simulink model "blocos"  (R2013a)
settings: Solver=ode45  StartTime=0.0  StopTime=3  RelTol=1e-3
values from neighbouring files (symbols this model uses):
  alpha = (Lms+Lls)    (= 0.11)    [Sugestao de estrutura de programa.m]
  beta = (Llr+Lms)    (= 0.11)    [Sugestao de estrutura de programa.m]
  Bm = dl    (= 0.0001)    [Sugestao de estrutura de programa.m]
  f = 60    [Sugestao de estrutura de programa.m]
  J = Jl    (= 0.002)    [Sugestao de estrutura de programa.m]
  Jl = 0.002    [Sugestao de estrutura de programa.m]
  Llr = 0.01    [Sugestao de estrutura de programa.m]
  Lls = 0.01    [Sugestao de estrutura de programa.m]
  Lms = 0.1    [Sugestao de estrutura de programa.m]
  P = 2    [Sugestao de estrutura de programa.m]
  polos = 2    [Sugestao de estrutura de programa.m]
  rrs = 1    [Sugestao de estrutura de programa.m]
  rs = 0.8    [Sugestao de estrutura de programa.m]
  thetar = 0.0    (= 0)    [Sugestao de estrutura de programa.m]
  U = 220    [Sugestao de estrutura de programa.m]
undefined symbols (not defined in the file or in its folder): i
settings Model: Creator=Charles  LastModifiedBy=Charles

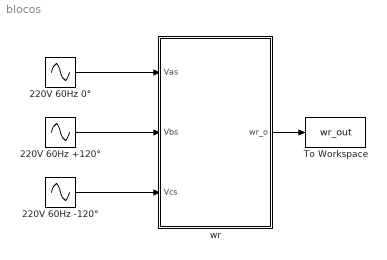
== system blocos ==
  220V 60Hz +120° : Sin  Amplitude=220  Frequency=377  Phase=2.0944  SampleTime=0
  220V 60Hz -120° : Sin  Amplitude=220  Frequency=377  Phase=-2.0944  SampleTime=0
  220V 60Hz 0° : Sin  Amplitude=220  Frequency=377  SampleTime=0
  To Workspace : ToWorkspace  VariableName=wr_out  SampleTime=-1  SaveFormat=Timeseries
  wr : Subsystem
  wires:
  220V 60Hz 0°/1 -> wr/1(Vas)
  wr/1(wr_o) -> To Workspace/1
  220V 60Hz +120°/1 -> wr/2(Vbs)
  220V 60Hz -120°/1 -> wr/3(Vcs)

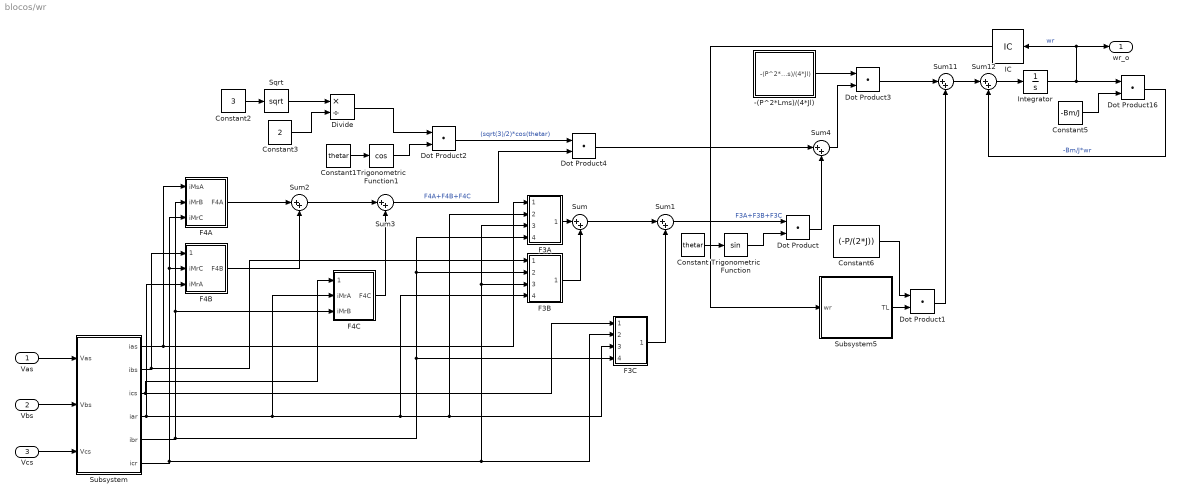
== system blocos/wr ==
  Vas : Inport
  Vbs : Inport  Port=2
  Vcs : Inport  Port=3
  -(P^2*Lms)/(4*Jl) : Subsystem
  Constant : Constant  Value=thetar
  Constant1 : Constant  Value=thetar
  Constant2 : Constant  Value=3
  Constant3 : Constant  Value=2
  Constant5 : Constant  Value=-Bm/J
  Constant6 : Constant  Value=(-P/(2*J))
  Divide : Product  Inputs=*/
  Dot Product{,1..4,16} (6 alike) : DotProduct  InputSameDT=on  OutDataTypeStr=Inherit: Inherit via internal rule
  F3A : Subsystem
  F3B : Subsystem
  F3C : Subsystem
  F4A : Subsystem
  F4B : Subsystem
  F4C : Subsystem
  IC : InitialCondition  Value=0.000001
  Integrator : Integrator
  Sqrt : Sqrt  SaturateOnIntegerOverflow=on
  Subsystem : Subsystem
  Subsystem5 : Subsystem
  Sum{,1..4,11..12} (7 alike) : Sum  Inputs=|++
  Trigonometric Function : Trigonometry
  Trigonometric Function1 : Trigonometry  Operator=cos
  wr_o : Outport
  wires:
  Dot Product16/1 -> Sum12/2  "-Bm/J*wr"
  Integrator/1 -> wr_o/1, IC/1, Dot Product16/1  "wr"
  Sum11/1 -> Sum12/1
  Constant5/1 -> Dot Product16/2
  Subsystem/3(ics) -> F3C/1(iMsC), F4C/1(iMsC)
  Subsystem/4(iar) -> F3C/3(iMrA), F3A/2(iMrA), F3B/4(iMrA), F4C/2(iMrA), F4B/3(iMrA)
  Subsystem/5(ibr) -> F3C/4(iMrB), F3B/2(iMrB), F3A/4(iMrB), F4C/3(iMrB), F4A/2(iMrB)
  Vbs/1 -> Subsystem/2(Vbs)
  Vcs/1 -> Subsystem/3(Vcs)
  Subsystem/2(ibs) -> F3B/1(iMsB), F4B/1(iMsB)
  Subsystem/6(icr) -> F3C/2(iMrC), F3B/3(iMrC), F3A/3(iMrC), F4B/2(iMrC), F4A/3(iMrC)
  Subsystem/1(ias) -> F3A/1(iMsA), F4A/1(iMsA)
  F4C/1(F4C) -> Sum3/2
  Sum3/1 -> Dot Product4/2  "F4A+F4B+F4C"
  Divide/1 -> Dot Product2/1
  Constant1/1 -> Trigonometric Function1/1
  F3B/1(F3B) -> Sum/2
  Trigonometric Function/1 -> Dot Product/2
  Constant2/1 -> Sqrt/1
  Sum1/1 -> Dot Product/1  "F3A+F3B+F3C"
  Dot Product4/1 -> Sum4/1
  F4B/1(F4B) -> Sum2/2
  F3C/1(F3C) -> Sum1/2
  Dot Product/1 -> Sum4/2
  Trigonometric Function1/1 -> Dot Product2/2
  Sum/1 -> Sum1/1
  Sqrt/1 -> Divide/1
  F4A/1(F4A) -> Sum2/1
  Sum2/1 -> Sum3/1
  Constant3/1 -> Divide/2
  Dot Product2/1 -> Dot Product4/1  "(sqrt(3)/2)*cos(thetar)"
  Dot Product3/1 -> Sum11/1
  -(P^2*Lms)/(4*Jl)/1(-(P^2*Lms)/(4*Jl)) -> Dot Product3/1
  Sum4/1 -> Dot Product3/2
  F3A/1(F3A) -> Sum/1
  Constant/1 -> Trigonometric Function/1
  Vas/1 -> Subsystem/1(Vas)
  Subsystem5/1(TL) -> Dot Product1/2
  Dot Product1/1 -> Sum11/2
  Constant6/1 -> Dot Product1/1
  Sum12/1 -> Integrator/1
  IC/1 -> Subsystem5/1(wr)

== system blocos/wr/-(P^2*Lms)//(4*Jl) ==
  Constant : Constant  Value=P
  Constant1 : Constant  Value=-Lms
  Constant2 : Constant  Value=4*Jl
  Divide : Product  Inputs=*/
  Dot Product : DotProduct  InputSameDT=on  OutDataTypeStr=Inherit: Inherit via internal rule
  Dot Product1 : DotProduct  InputSameDT=on  OutDataTypeStr=Inherit: Inherit via internal rule
  -(P^2*Lms)/(4*Jl) : Outport
  wires:
  Divide/1 -> -(P^2*Lms)/(4*Jl)/1  "-(P^2*Lms)/(4*Jl)"
  Constant2/1 -> Divide/2
  Dot Product1/1 -> Divide/1  "-P^2*Lms"
  Dot Product/1 -> Dot Product1/1  "P^2"
  Constant1/1 -> Dot Product1/2
  Constant/1 -> Dot Product/2, Dot Product/1

== system blocos/wr/F3A ==
  iMsA : Inport
  iMrA : Inport  Port=2
  iMrC : Inport  Port=3
  iMrB : Inport  Port=4
  Constant : Constant  Value=-0.5
  Dot Product : DotProduct  InputSameDT=on  OutDataTypeStr=Inherit: Inherit via internal rule
  Dot Product1 : DotProduct  InputSameDT=on  OutDataTypeStr=Inherit: Inherit via internal rule
  Dot Product2 : DotProduct  InputSameDT=on  OutDataTypeStr=Inherit: Inherit via internal rule
  Sum : Sum  Inputs=|++
  Sum1 : Sum  Inputs=|++
  F3A : Outport
  wires:
  iMrB/1 -> Dot Product/1
  Sum1/1 -> Dot Product2/1  "iMrA-0.5*iMrB-0.5*iMrC"
  iMrA/1 -> Sum1/2
  Dot Product2/1 -> F3A/1
  iMrC/1 -> Dot Product1/1
  Constant/1 -> Dot Product/2, Dot Product1/2
  Dot Product/1 -> Sum/1  "-0.5*iMrB"
  Sum/1 -> Sum1/1  "-0.5*iMrB-0.5*iMrC"
  iMsA/1 -> Dot Product2/2
  Dot Product1/1 -> Sum/2  "-0.5*iMrC"

== system blocos/wr/F3B ==
  iMsB : Inport
  iMrB : Inport  Port=2
  iMrC : Inport  Port=3
  iMrA : Inport  Port=4
  Constant : Constant  Value=-0.5
  Dot Product : DotProduct  InputSameDT=on  OutDataTypeStr=Inherit: Inherit via internal rule
  Dot Product1 : DotProduct  InputSameDT=on  OutDataTypeStr=Inherit: Inherit via internal rule
  Dot Product2 : DotProduct  InputSameDT=on  OutDataTypeStr=Inherit: Inherit via internal rule
  Sum : Sum  Inputs=|++
  Sum1 : Sum  Inputs=|++
  F3B : Outport
  wires:
  iMrA/1 -> Dot Product/1
  Sum1/1 -> Dot Product2/1  "iMrB-0.5*iMrA-0.5*iMrC"
  iMrB/1 -> Sum1/2
  Dot Product2/1 -> F3B/1
  iMrC/1 -> Dot Product1/1
  Constant/1 -> Dot Product/2, Dot Product1/2
  Dot Product/1 -> Sum/1  "-0.5*iMrA"
  Sum/1 -> Sum1/1  "-0.5*iMrA-0.5*iMrC"
  iMsB/1 -> Dot Product2/2
  Dot Product1/1 -> Sum/2  "-0.5*iMrC"

== system blocos/wr/F3C ==
  iMsC : Inport
  iMrC : Inport  Port=2
  iMrA : Inport  Port=3
  iMrB : Inport  Port=4
  Constant : Constant  Value=-0.5
  Dot Product : DotProduct  InputSameDT=on  OutDataTypeStr=Inherit: Inherit via internal rule
  Dot Product1 : DotProduct  InputSameDT=on  OutDataTypeStr=Inherit: Inherit via internal rule
  Dot Product2 : DotProduct  InputSameDT=on  OutDataTypeStr=Inherit: Inherit via internal rule
  Sum : Sum  Inputs=|++
  Sum1 : Sum  Inputs=|++
  F3C : Outport
  wires:
  iMrB/1 -> Dot Product/1
  Sum1/1 -> Dot Product2/1  "iMrC-0.5*iMrB-0.5*iMrA"
  iMrC/1 -> Sum1/2
  Dot Product2/1 -> F3C/1
  iMrA/1 -> Dot Product1/1
  Constant/1 -> Dot Product/2, Dot Product1/2
  Dot Product/1 -> Sum/1  "-0.5*iMrB"
  Sum/1 -> Sum1/1  "-0.5*iMrB-0.5*iMrA"
  iMsC/1 -> Dot Product2/2
  Dot Product1/1 -> Sum/2  "-0.5*iMrA"

== system blocos/wr/F4A ==
  iMsA : Inport
  iMrB : Inport  Port=2
  iMrC : Inport  Port=3
  Dot Product : DotProduct  InputSameDT=on  OutDataTypeStr=Inherit: Inherit via internal rule
  Subtract1 : Sum  Inputs=+-
  F4A : Outport
  wires:
  Subtract1/1 -> Dot Product/2
  iMrC/1 -> Subtract1/2
  iMrB/1 -> Subtract1/1
  Dot Product/1 -> F4A/1
  iMsA/1 -> Dot Product/1

== system blocos/wr/F4B ==
  iMsB : Inport
  iMrC : Inport  Port=2
  iMrA : Inport  Port=3
  Dot Product : DotProduct  InputSameDT=on  OutDataTypeStr=Inherit: Inherit via internal rule
  Subtract1 : Sum  Inputs=+-
  F4B : Outport
  wires:
  Subtract1/1 -> Dot Product/2
  iMrA/1 -> Subtract1/2
  iMrC/1 -> Subtract1/1
  Dot Product/1 -> F4B/1
  iMsB/1 -> Dot Product/1

== system blocos/wr/F4C ==
  iMsC : Inport
  iMrA : Inport  Port=2
  iMrB : Inport  Port=3
  Dot Product : DotProduct  InputSameDT=on  OutDataTypeStr=Inherit: Inherit via internal rule
  Subtract1 : Sum  Inputs=+-
  F4C : Outport
  wires:
  Subtract1/1 -> Dot Product/2
  iMrB/1 -> Subtract1/2
  iMrA/1 -> Subtract1/1
  Dot Product/1 -> F4C/1
  iMsC/1 -> Dot Product/1

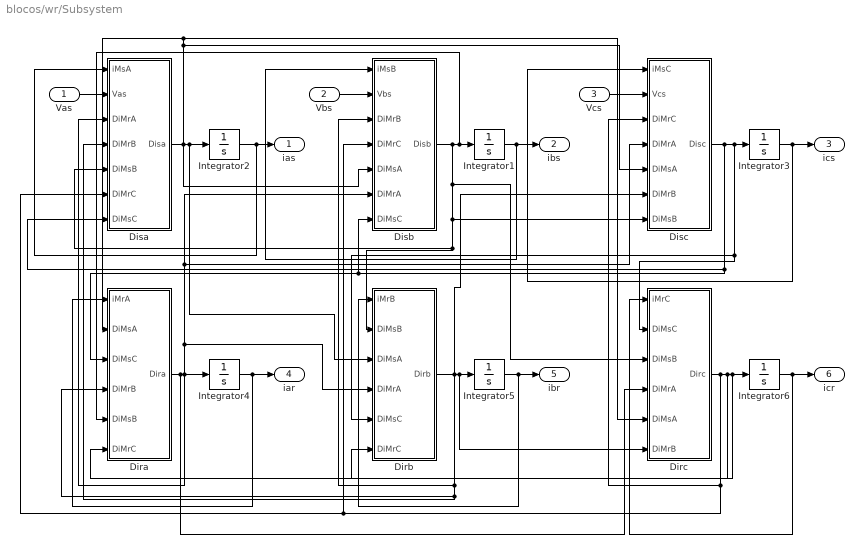
== system blocos/wr/Subsystem ==
  Vas : Inport
  Vbs : Inport  Port=2
  Vcs : Inport  Port=3
  Dira : Subsystem
  Dirb : Subsystem
  Dirc : Subsystem
  Disa : Subsystem
  Disb : Subsystem
  Disc : Subsystem
  Integrator{1..6} (6 alike) : Integrator
  ias : Outport
  ibs : Outport  Port=2
  ics : Outport  Port=3
  iar : Outport  Port=4
  ibr : Outport  Port=5
  icr : Outport  Port=6
  wires:
  Integrator2/1 -> Disa/1(iMsA), ias/1
  Disa/1(Disa) -> Dira/2(DiMsA), Dirc/5(DiMsA), Disc/5(DiMsA), Disb/5(DiMsA), Dirb/3(DiMsA), Integrator2/1
  Integrator1/1 -> Disb/1(iMsB), ibs/1
  Disb/1(Disb) -> Dirc/3(DiMsB), Dirb/2(DiMsB), Disa/5(DiMsB), Disc/7(DiMsB), Dira/5(DiMsB), Integrator1/1
  Integrator3/1 -> Disc/1(iMsC), ics/1
  Disc/1(Disc) -> Dira/3(DiMsC), Disb/7(DiMsC), Disa/7(DiMsC), Dirc/2(DiMsC), Dirb/5(DiMsC), Integrator3/1
  Integrator4/1 -> Dira/1(iMrA), iar/1
  Dira/1(Dira) -> Dirc/4(DiMrA), Dirb/4(DiMrA), Disc/4(DiMrA), Disb/6(DiMrA), Disa/3(DiMrA), Integrator4/1
  Integrator5/1 -> Dirb/1(iMrB), ibr/1
  Dirb/1(Dirb) -> Dira/4(DiMrB), Disa/4(DiMrB), Disb/3(DiMrB), Disc/6(DiMrB), Dirc/6(DiMrB), Integrator5/1
  Integrator6/1 -> Dirc/1(iMrC), icr/1
  Dirc/1(Dirc) -> Disc/3(DiMrC), Disb/4(DiMrC), Disa/6(DiMrC), Dirb/6(DiMrC), Dira/6(DiMrC), Integrator6/1
  Vas/1 -> Disa/2(Vas)
  Vbs/1 -> Disb/2(Vbs)
  Vcs/1 -> Disc/2(Vcs)

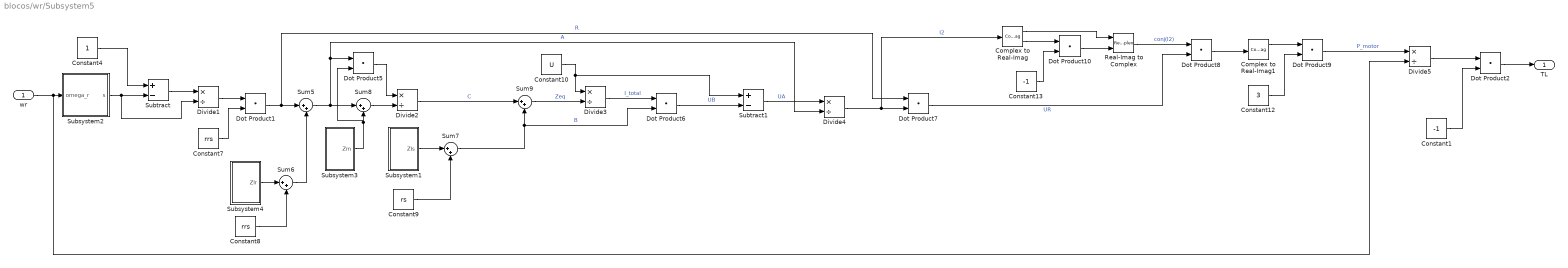
== system blocos/wr/Subsystem5 ==
  wr : Inport
  Complex to Real-Imag : ComplexToRealImag
  Complex to Real-Imag1 : ComplexToRealImag
  Constant1 : Constant  Value=-1
  Constant10 : Constant  Value=U
  Constant12 : Constant  Value=3
  Constant13 : Constant  Value=-1
  Constant4 : Constant
  Constant7 : Constant  Value=rrs
  Constant8 : Constant  Value=rrs
  Constant9 : Constant  Value=rs
  Divide{1..5} (5 alike) : Product  Inputs=*/
  Dot Product{1..2,5..10} (8 alike) : DotProduct  InputSameDT=on  OutDataTypeStr=Inherit: Inherit via internal rule
  Real-Imag to Complex : RealImagToComplex
  Subsystem1 : Subsystem
  Subsystem2 : Subsystem
  Subsystem3 : Subsystem
  Subsystem4 : Subsystem
  Subtract : Sum  Inputs=+-
  Subtract1 : Sum  Inputs=+-
  Sum{5..9} (5 alike) : Sum  Inputs=|++
  TL : Outport
  wires:
  Constant7/1 -> Dot Product1/2
  Dot Product1/1 -> Dot Product7/1, Sum5/1  "R"
  Divide1/1 -> Dot Product1/1
  Constant4/1 -> Subtract/1
  Subtract/1 -> Divide1/1
  Subsystem2/1(s) -> Divide1/2, Subtract/2
  wr/1 -> Divide5/2, Subsystem2/1(omega_r)
  Constant10/1 -> Subtract1/1, Divide3/1
  Subsystem3/1(Zm) -> Dot Product5/2, Sum8/2
  Divide3/1 -> Dot Product6/1  "I_total"
  Subtract1/1 -> Divide4/1  "UA"
  Sum8/1 -> Divide2/2
  Sum6/1 -> Sum5/2
  Constant8/1 -> Sum6/2
  Sum5/1 -> Divide4/2, Dot Product5/1, Sum8/1  "A"
  Divide4/1 -> Complex to Real-Imag/1, Dot Product7/2  "I2"
  Subsystem4/1(Zlr) -> Sum6/1
  Divide2/1 -> Sum9/1  "C"
  Dot Product5/1 -> Divide2/1
  Dot Product7/1 -> Dot Product8/2  "UR"
  Subsystem1/1(Zls) -> Sum7/1
  Constant9/1 -> Sum7/2
  Dot Product6/1 -> Subtract1/2  "UB"
  Sum7/1 -> Dot Product6/2, Sum9/2  "B"
  Sum9/1 -> Divide3/2  "Zeq"
  Constant12/1 -> Dot Product9/2
  Complex to Real-Imag/2 -> Dot Product10/1
  Complex to Real-Imag1/1 -> Dot Product9/1
  Dot Product9/1 -> Divide5/1  "P_motor"
  Complex to Real-Imag/1 -> Real-Imag to Complex/1
  Dot Product10/1 -> Real-Imag to Complex/2
  Constant13/1 -> Dot Product10/2
  Real-Imag to Complex/1 -> Dot Product8/1  "conj(I2)"
  Dot Product8/1 -> Complex to Real-Imag1/1
  Constant1/1 -> Dot Product2/2
  Divide5/1 -> Dot Product2/1
  Dot Product2/1 -> TL/1

== system blocos/wr/Subsystem/Dira ==
  iMrA : Inport
  DiMsA : Inport  Port=2
  DiMsC : Inport  Port=3
  DiMrB : Inport  Port=4
  DiMsB : Inport  Port=5
  DiMrC : Inport  Port=6
  1/beta : Constant  Value=1/beta
  Constant : Constant  Value=-rrs
  Dot Product : DotProduct  InputSameDT=on  OutDataTypeStr=Inherit: Inherit via internal rule
  Dot Product1 : DotProduct  InputSameDT=on  OutDataTypeStr=Inherit: Inherit via internal rule
  F1A1 : Subsystem
  F2A 1 : Subsystem
  Sum1 : Sum  Inputs=|++
  Sum2 : Sum  Inputs=|++
  Dira : Outport
  wires:
  Dot Product/1 -> Sum1/1  "-rrs*iMrA"
  iMrA/1 -> Dot Product/1
  Constant/1 -> Dot Product/2
  Sum1/1 -> Sum2/1  "-rrs*iMrA+F1Ar"
  Sum2/1 -> Dot Product1/1  "-rrs*iMrA+F1Ar+F2Ar"
  F2A 1/1(F2Ar) -> Sum2/2
  DiMrC/1 -> F1A1/2(DiMrC)
  F1A1/1(F1Ar) -> Sum1/2
  DiMrB/1 -> F1A1/1(DiMrB)
  1/beta/1 -> Dot Product1/2
  DiMsB/1 -> F2A 1/3(DiMsB)
  Dot Product1/1 -> Dira/1
  DiMsC/1 -> F2A 1/2(DiMsC)
  DiMsA/1 -> F2A 1/1(DiMsA)

== system blocos/wr/Subsystem/Dirb ==
  iMrB : Inport
  DiMsB : Inport  Port=2
  DiMsA : Inport  Port=3
  DiMrA : Inport  Port=4
  DiMsC : Inport  Port=5
  DiMrC : Inport  Port=6
  1/beta : Constant  Value=1/beta
  Constant : Constant  Value=-rrs
  Dot Product : DotProduct  InputSameDT=on  OutDataTypeStr=Inherit: Inherit via internal rule
  Dot Product1 : DotProduct  InputSameDT=on  OutDataTypeStr=Inherit: Inherit via internal rule
  F1A1 : Subsystem
  F2A 1 : Subsystem
  Sum1 : Sum  Inputs=|++
  Sum2 : Sum  Inputs=|++
  Dirb : Outport
  wires:
  Dot Product/1 -> Sum1/1  "-rrs*iMrB"
  iMrB/1 -> Dot Product/1
  Constant/1 -> Dot Product/2
  Sum1/1 -> Sum2/1  "-rrs*iMrB+F1Br"
  Sum2/1 -> Dot Product1/1  "-rrs*iMrB+F1Br+F2Br"
  F2A 1/1(F2Br) -> Sum2/2
  DiMrC/1 -> F1A1/2(DiMrC)
  F1A1/1(F1Br) -> Sum1/2
  DiMrA/1 -> F1A1/1(DiMrA)
  1/beta/1 -> Dot Product1/2
  DiMsC/1 -> F2A 1/3(DiMsC)
  Dot Product1/1 -> Dirb/1
  DiMsA/1 -> F2A 1/2(DiMsA)
  DiMsB/1 -> F2A 1/1(DiMsB)

== system blocos/wr/Subsystem/Dirc ==
  iMrC : Inport
  DiMsC : Inport  Port=2
  DiMsB : Inport  Port=3
  DiMrA : Inport  Port=4
  DiMsA : Inport  Port=5
  DiMrB : Inport  Port=6
  1/beta : Constant  Value=1/beta
  Constant : Constant  Value=-rrs
  Dot Product : DotProduct  InputSameDT=on  OutDataTypeStr=Inherit: Inherit via internal rule
  Dot Product1 : DotProduct  InputSameDT=on  OutDataTypeStr=Inherit: Inherit via internal rule
  F1A1 : Subsystem
  F2A 1 : Subsystem
  Sum1 : Sum  Inputs=|++
  Sum2 : Sum  Inputs=|++
  Dirc : Outport
  wires:
  Dot Product/1 -> Sum1/1  "-rrs*iMrC"
  iMrC/1 -> Dot Product/1
  Constant/1 -> Dot Product/2
  Sum1/1 -> Sum2/1  "-rrs*iMrC+F1Cr"
  Sum2/1 -> Dot Product1/1  "-rrs*iMrC+F1Cr+F2Cr"
  F2A 1/1(F2Cr) -> Sum2/2
  DiMrB/1 -> F1A1/2(DiMrB)
  F1A1/1(F1Cr) -> Sum1/2
  DiMrA/1 -> F1A1/1(DiMrA)
  1/beta/1 -> Dot Product1/2
  DiMsA/1 -> F2A 1/3(DiMsA)
  Dot Product1/1 -> Dirc/1
  DiMsB/1 -> F2A 1/2(DiMsB)
  DiMsC/1 -> F2A 1/1(DiMsC)

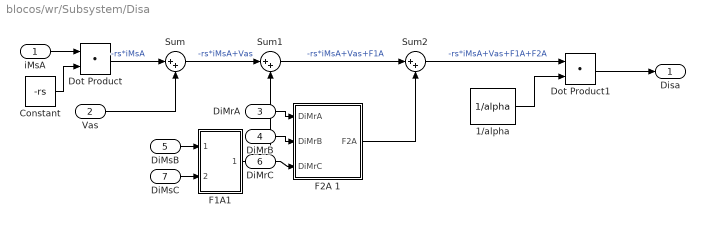
== system blocos/wr/Subsystem/Disa ==
  iMsA : Inport
  Vas : Inport  Port=2
  DiMrA : Inport  Port=3
  DiMrB : Inport  Port=4
  DiMsB : Inport  Port=5
  DiMrC : Inport  Port=6
  DiMsC : Inport  Port=7
  1/alpha : Constant  Value=1/alpha
  Constant : Constant  Value=-rs
  Dot Product : DotProduct  InputSameDT=on  OutDataTypeStr=Inherit: Inherit via internal rule
  Dot Product1 : DotProduct  InputSameDT=on  OutDataTypeStr=Inherit: Inherit via internal rule
  F1A1 : Subsystem
  F2A 1 : Subsystem
  Sum : Sum  Inputs=|++
  Sum1 : Sum  Inputs=|++
  Sum2 : Sum  Inputs=|++
  Disa : Outport
  wires:
  Dot Product/1 -> Sum/1  "-rs*iMsA"
  iMsA/1 -> Dot Product/1
  Constant/1 -> Dot Product/2
  Sum1/1 -> Sum2/1  "-rs*iMsA+Vas+F1A"
  Sum2/1 -> Dot Product1/1  "-rs*iMsA+Vas+F1A+F2A"
  Sum/1 -> Sum1/1  "-rs*iMsA+Vas"
  F2A 1/1(F2A) -> Sum2/2
  DiMsC/1 -> F1A1/2(DiMsC)
  F1A1/1(F1A) -> Sum1/2
  DiMsB/1 -> F1A1/1(DiMsB)
  1/alpha/1 -> Dot Product1/2
  DiMrC/1 -> F2A 1/3(DiMrC)
  Dot Product1/1 -> Disa/1
  Vas/1 -> Sum/2
  DiMrB/1 -> F2A 1/2(DiMrB)
  DiMrA/1 -> F2A 1/1(DiMrA)

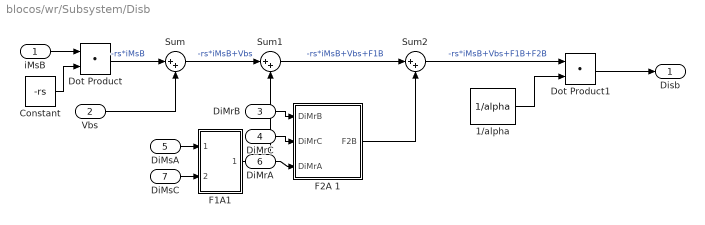
== system blocos/wr/Subsystem/Disb ==
  iMsB : Inport
  Vbs : Inport  Port=2
  DiMrB : Inport  Port=3
  DiMrC : Inport  Port=4
  DiMsA : Inport  Port=5
  DiMrA : Inport  Port=6
  DiMsC : Inport  Port=7
  1/alpha : Constant  Value=1/alpha
  Constant : Constant  Value=-rs
  Dot Product : DotProduct  InputSameDT=on  OutDataTypeStr=Inherit: Inherit via internal rule
  Dot Product1 : DotProduct  InputSameDT=on  OutDataTypeStr=Inherit: Inherit via internal rule
  F1A1 : Subsystem
  F2A 1 : Subsystem
  Sum : Sum  Inputs=|++
  Sum1 : Sum  Inputs=|++
  Sum2 : Sum  Inputs=|++
  Disb : Outport
  wires:
  Dot Product/1 -> Sum/1  "-rs*iMsB"
  iMsB/1 -> Dot Product/1
  Constant/1 -> Dot Product/2
  Sum1/1 -> Sum2/1  "-rs*iMsB+Vbs+F1B"
  Sum2/1 -> Dot Product1/1  "-rs*iMsB+Vbs+F1B+F2B"
  Sum/1 -> Sum1/1  "-rs*iMsB+Vbs"
  F2A 1/1(F2B) -> Sum2/2
  DiMsC/1 -> F1A1/2(DiMsC)
  F1A1/1(F1B) -> Sum1/2
  DiMsA/1 -> F1A1/1(DiMsA)
  1/alpha/1 -> Dot Product1/2
  DiMrA/1 -> F2A 1/3(DiMrA)
  Dot Product1/1 -> Disb/1
  Vbs/1 -> Sum/2
  DiMrC/1 -> F2A 1/2(DiMrC)
  DiMrB/1 -> F2A 1/1(DiMrB)

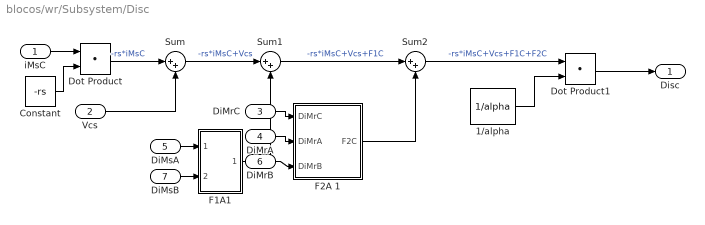
== system blocos/wr/Subsystem/Disc ==
  iMsC : Inport
  Vcs : Inport  Port=2
  DiMrC : Inport  Port=3
  DiMrA : Inport  Port=4
  DiMsA : Inport  Port=5
  DiMrB : Inport  Port=6
  DiMsB : Inport  Port=7
  1/alpha : Constant  Value=1/alpha
  Constant : Constant  Value=-rs
  Dot Product : DotProduct  InputSameDT=on  OutDataTypeStr=Inherit: Inherit via internal rule
  Dot Product1 : DotProduct  InputSameDT=on  OutDataTypeStr=Inherit: Inherit via internal rule
  F1A1 : Subsystem
  F2A 1 : Subsystem
  Sum : Sum  Inputs=|++
  Sum1 : Sum  Inputs=|++
  Sum2 : Sum  Inputs=|++
  Disc : Outport
  wires:
  Dot Product/1 -> Sum/1  "-rs*iMsC"
  iMsC/1 -> Dot Product/1
  Constant/1 -> Dot Product/2
  Sum1/1 -> Sum2/1  "-rs*iMsC+Vcs+F1C"
  Sum2/1 -> Dot Product1/1  "-rs*iMsC+Vcs+F1C+F2C"
  Sum/1 -> Sum1/1  "-rs*iMsC+Vcs"
  F2A 1/1(F2C) -> Sum2/2
  DiMsB/1 -> F1A1/2(DiMsB)
  F1A1/1(F1C) -> Sum1/2
  DiMsA/1 -> F1A1/1(DiMsA)
  1/alpha/1 -> Dot Product1/2
  DiMrB/1 -> F2A 1/3(DiMrB)
  Dot Product1/1 -> Disc/1
  Vcs/1 -> Sum/2
  DiMrA/1 -> F2A 1/2(DiMrA)
  DiMrC/1 -> F2A 1/1(DiMrC)

== system blocos/wr/Subsystem5/Subsystem1 ==
  Constant10 : Constant  Value=f
  Constant11 : Constant  Value=pi
  Constant12 : Constant  Value=2
  Constant13 : Constant  Value=i
  Constant9 : Constant  Value=Lls
  Dot Product{5..8} (4 alike) : DotProduct  InputSameDT=on  OutDataTypeStr=Inherit: Inherit via internal rule
  Zls : Outport
  wires:
  Constant13/1 -> Dot Product8/2
  Dot Product7/1 -> Dot Product6/1
  Constant9/1 -> Dot Product5/2
  Constant12/1 -> Dot Product8/1
  Dot Product8/1 -> Dot Product7/1
  Constant10/1 -> Dot Product6/2
  Dot Product5/1 -> Zls/1
  Dot Product6/1 -> Dot Product5/1
  Constant11/1 -> Dot Product7/2

== system blocos/wr/Subsystem5/Subsystem2 ==
  omega_r : Inport
  Divide1 : Product  Inputs=*/
  Subsystem1 : Subsystem
  Subtract : Sum  Inputs=+-
  s : Outport
  wires:
  omega_r/1 -> Subtract/2
  Subtract/1 -> Divide1/1
  Divide1/1 -> s/1
  Subsystem1/1(omega_1) -> Divide1/2, Subtract/1

== system blocos/wr/Subsystem5/Subsystem3 ==
  Constant10 : Constant  Value=f
  Constant11 : Constant  Value=pi
  Constant12 : Constant  Value=2
  Constant13 : Constant  Value=i
  Constant9 : Constant  Value=Lms
  Dot Product{5..8} (4 alike) : DotProduct  InputSameDT=on  OutDataTypeStr=Inherit: Inherit via internal rule
  Zm : Outport
  wires:
  Constant13/1 -> Dot Product8/2
  Dot Product7/1 -> Dot Product6/1
  Constant9/1 -> Dot Product5/2
  Constant12/1 -> Dot Product8/1
  Dot Product8/1 -> Dot Product7/1
  Constant10/1 -> Dot Product6/2
  Dot Product5/1 -> Zm/1
  Dot Product6/1 -> Dot Product5/1
  Constant11/1 -> Dot Product7/2

== system blocos/wr/Subsystem5/Subsystem4 ==
  Constant10 : Constant  Value=f
  Constant11 : Constant  Value=pi
  Constant12 : Constant  Value=2
  Constant13 : Constant  Value=i
  Constant9 : Constant  Value=Llr
  Dot Product{5..8} (4 alike) : DotProduct  InputSameDT=on  OutDataTypeStr=Inherit: Inherit via internal rule
  Zlr : Outport
  wires:
  Constant13/1 -> Dot Product8/2
  Dot Product7/1 -> Dot Product6/1
  Constant9/1 -> Dot Product5/2
  Constant12/1 -> Dot Product8/1
  Dot Product8/1 -> Dot Product7/1
  Constant10/1 -> Dot Product6/2
  Dot Product5/1 -> Zlr/1
  Dot Product6/1 -> Dot Product5/1
  Constant11/1 -> Dot Product7/2

== system blocos/wr/Subsystem/Dira/F1A1 ==
  DiMrB : Inport
  DiMrC : Inport  Port=2
  Constant : Constant  Value=Lms/2
  Dot Product : DotProduct  InputSameDT=on  OutDataTypeStr=Inherit: Inherit via internal rule
  Sum : Sum  Inputs=|++
  F1Ar : Outport
  wires:
  Constant/1 -> Dot Product/1
  Dot Product/1 -> F1Ar/1
  Sum/1 -> Dot Product/2
  DiMrC/1 -> Sum/2
  DiMrB/1 -> Sum/1

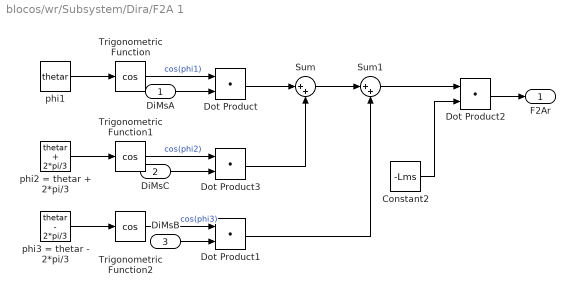
== system blocos/wr/Subsystem/Dira/F2A 1 ==
  DiMsA : Inport
  DiMsC : Inport  Port=2
  DiMsB : Inport  Port=3
  Constant2 : Constant  Value=-Lms
  Dot Product{,1..3} (4 alike) : DotProduct  InputSameDT=on  OutDataTypeStr=Inherit: Inherit via internal rule
  Sum : Sum  Inputs=|++
  Sum1 : Sum  Inputs=|++
  Trigonometric Function : Trigonometry  Operator=cos
  Trigonometric Function1 : Trigonometry  Operator=cos
  Trigonometric Function2 : Trigonometry  Operator=cos
  phi1 : Constant  Value=thetar
  phi2 = thetar + 2*pi/3 : Constant  Value=thetar + 2*pi/3
  phi3 = thetar - 2*pi/3 : Constant  Value=thetar - 2*pi/3
  F2Ar : Outport
  wires:
  Dot Product2/1 -> F2Ar/1
  Constant2/1 -> Dot Product2/2
  DiMsB/1 -> Dot Product1/2
  DiMsA/1 -> Dot Product/2
  phi1/1 -> Trigonometric Function/1
  Trigonometric Function2/1 -> Dot Product1/1  "cos(phi3)"
  phi2 = thetar + 2*pi/3/1 -> Trigonometric Function1/1
  Trigonometric Function/1 -> Dot Product/1  "cos(phi1)"
  phi3 = thetar - 2*pi/3/1 -> Trigonometric Function2/1
  Trigonometric Function1/1 -> Dot Product3/1  "cos(phi2)"
  Sum1/1 -> Dot Product2/1
  DiMsC/1 -> Dot Product3/2
  Dot Product1/1 -> Sum1/2
  Dot Product3/1 -> Sum/2
  Dot Product/1 -> Sum/1
  Sum/1 -> Sum1/1

== system blocos/wr/Subsystem/Dirb/F1A1 ==
  DiMrA : Inport
  DiMrC : Inport  Port=2
  Constant : Constant  Value=Lms/2
  Dot Product : DotProduct  InputSameDT=on  OutDataTypeStr=Inherit: Inherit via internal rule
  Sum : Sum  Inputs=|++
  F1Br : Outport
  wires:
  Constant/1 -> Dot Product/1
  Dot Product/1 -> F1Br/1
  Sum/1 -> Dot Product/2
  DiMrC/1 -> Sum/2
  DiMrA/1 -> Sum/1

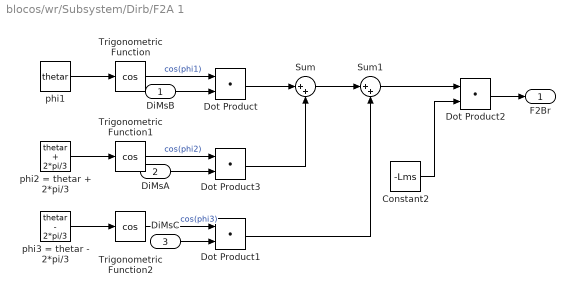
== system blocos/wr/Subsystem/Dirb/F2A 1 ==
  DiMsB : Inport
  DiMsA : Inport  Port=2
  DiMsC : Inport  Port=3
  Constant2 : Constant  Value=-Lms
  Dot Product{,1..3} (4 alike) : DotProduct  InputSameDT=on  OutDataTypeStr=Inherit: Inherit via internal rule
  Sum : Sum  Inputs=|++
  Sum1 : Sum  Inputs=|++
  Trigonometric Function : Trigonometry  Operator=cos
  Trigonometric Function1 : Trigonometry  Operator=cos
  Trigonometric Function2 : Trigonometry  Operator=cos
  phi1 : Constant  Value=thetar
  phi2 = thetar + 2*pi/3 : Constant  Value=thetar + 2*pi/3
  phi3 = thetar - 2*pi/3 : Constant  Value=thetar - 2*pi/3
  F2Br : Outport
  wires:
  Dot Product2/1 -> F2Br/1
  Constant2/1 -> Dot Product2/2
  DiMsC/1 -> Dot Product1/2
  DiMsB/1 -> Dot Product/2
  phi1/1 -> Trigonometric Function/1
  Trigonometric Function2/1 -> Dot Product1/1  "cos(phi3)"
  phi2 = thetar + 2*pi/3/1 -> Trigonometric Function1/1
  Trigonometric Function/1 -> Dot Product/1  "cos(phi1)"
  phi3 = thetar - 2*pi/3/1 -> Trigonometric Function2/1
  Trigonometric Function1/1 -> Dot Product3/1  "cos(phi2)"
  Sum1/1 -> Dot Product2/1
  DiMsA/1 -> Dot Product3/2
  Dot Product1/1 -> Sum1/2
  Dot Product3/1 -> Sum/2
  Dot Product/1 -> Sum/1
  Sum/1 -> Sum1/1

== system blocos/wr/Subsystem/Dirc/F1A1 ==
  DiMrA : Inport
  DiMrB : Inport  Port=2
  Constant : Constant  Value=Lms/2
  Dot Product : DotProduct  InputSameDT=on  OutDataTypeStr=Inherit: Inherit via internal rule
  Sum : Sum  Inputs=|++
  F1Cr : Outport
  wires:
  Constant/1 -> Dot Product/1
  Dot Product/1 -> F1Cr/1
  Sum/1 -> Dot Product/2
  DiMrB/1 -> Sum/2
  DiMrA/1 -> Sum/1

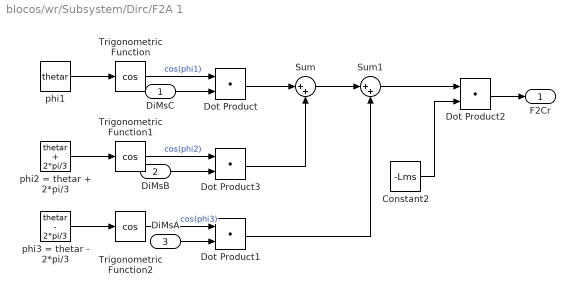
== system blocos/wr/Subsystem/Dirc/F2A 1 ==
  DiMsC : Inport
  DiMsB : Inport  Port=2
  DiMsA : Inport  Port=3
  Constant2 : Constant  Value=-Lms
  Dot Product{,1..3} (4 alike) : DotProduct  InputSameDT=on  OutDataTypeStr=Inherit: Inherit via internal rule
  Sum : Sum  Inputs=|++
  Sum1 : Sum  Inputs=|++
  Trigonometric Function : Trigonometry  Operator=cos
  Trigonometric Function1 : Trigonometry  Operator=cos
  Trigonometric Function2 : Trigonometry  Operator=cos
  phi1 : Constant  Value=thetar
  phi2 = thetar + 2*pi/3 : Constant  Value=thetar + 2*pi/3
  phi3 = thetar - 2*pi/3 : Constant  Value=thetar - 2*pi/3
  F2Cr : Outport
  wires:
  Dot Product2/1 -> F2Cr/1
  Constant2/1 -> Dot Product2/2
  DiMsA/1 -> Dot Product1/2
  DiMsC/1 -> Dot Product/2
  phi1/1 -> Trigonometric Function/1
  Trigonometric Function2/1 -> Dot Product1/1  "cos(phi3)"
  phi2 = thetar + 2*pi/3/1 -> Trigonometric Function1/1
  Trigonometric Function/1 -> Dot Product/1  "cos(phi1)"
  phi3 = thetar - 2*pi/3/1 -> Trigonometric Function2/1
  Trigonometric Function1/1 -> Dot Product3/1  "cos(phi2)"
  Sum1/1 -> Dot Product2/1
  DiMsB/1 -> Dot Product3/2
  Dot Product1/1 -> Sum1/2
  Dot Product3/1 -> Sum/2
  Dot Product/1 -> Sum/1
  Sum/1 -> Sum1/1

== system blocos/wr/Subsystem/Disa/F1A1 ==
  DiMsB : Inport
  DiMsC : Inport  Port=2
  Constant : Constant  Value=Lms/2
  Dot Product : DotProduct  InputSameDT=on  OutDataTypeStr=Inherit: Inherit via internal rule
  Sum : Sum  Inputs=|++
  F1A : Outport
  wires:
  Constant/1 -> Dot Product/1
  Dot Product/1 -> F1A/1
  Sum/1 -> Dot Product/2
  DiMsC/1 -> Sum/2
  DiMsB/1 -> Sum/1

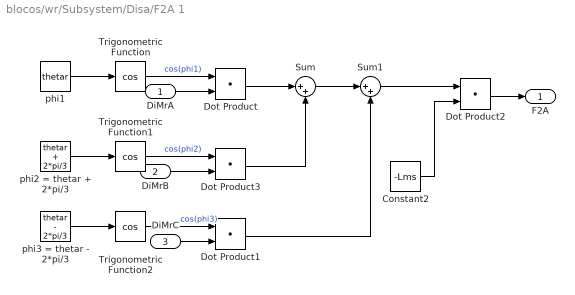
== system blocos/wr/Subsystem/Disa/F2A 1 ==
  DiMrA : Inport
  DiMrB : Inport  Port=2
  DiMrC : Inport  Port=3
  Constant2 : Constant  Value=-Lms
  Dot Product{,1..3} (4 alike) : DotProduct  InputSameDT=on  OutDataTypeStr=Inherit: Inherit via internal rule
  Sum : Sum  Inputs=|++
  Sum1 : Sum  Inputs=|++
  Trigonometric Function : Trigonometry  Operator=cos
  Trigonometric Function1 : Trigonometry  Operator=cos
  Trigonometric Function2 : Trigonometry  Operator=cos
  phi1 : Constant  Value=thetar
  phi2 = thetar + 2*pi/3 : Constant  Value=thetar + 2*pi/3
  phi3 = thetar - 2*pi/3 : Constant  Value=thetar - 2*pi/3
  F2A : Outport
  wires:
  Dot Product2/1 -> F2A/1
  Constant2/1 -> Dot Product2/2
  DiMrC/1 -> Dot Product1/2
  DiMrA/1 -> Dot Product/2
  phi1/1 -> Trigonometric Function/1
  Trigonometric Function2/1 -> Dot Product1/1  "cos(phi3)"
  phi2 = thetar + 2*pi/3/1 -> Trigonometric Function1/1
  Trigonometric Function/1 -> Dot Product/1  "cos(phi1)"
  phi3 = thetar - 2*pi/3/1 -> Trigonometric Function2/1
  Trigonometric Function1/1 -> Dot Product3/1  "cos(phi2)"
  Sum1/1 -> Dot Product2/1
  DiMrB/1 -> Dot Product3/2
  Dot Product1/1 -> Sum1/2
  Dot Product3/1 -> Sum/2
  Dot Product/1 -> Sum/1
  Sum/1 -> Sum1/1

== system blocos/wr/Subsystem/Disb/F1A1 ==
  DiMsA : Inport
  DiMsC : Inport  Port=2
  Constant : Constant  Value=Lms/2
  Dot Product : DotProduct  InputSameDT=on  OutDataTypeStr=Inherit: Inherit via internal rule
  Sum : Sum  Inputs=|++
  F1B : Outport
  wires:
  Constant/1 -> Dot Product/1
  Dot Product/1 -> F1B/1
  Sum/1 -> Dot Product/2
  DiMsC/1 -> Sum/2
  DiMsA/1 -> Sum/1

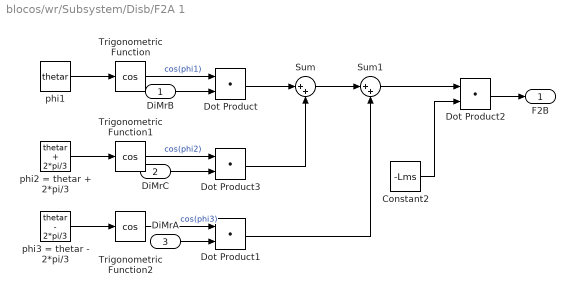
== system blocos/wr/Subsystem/Disb/F2A 1 ==
  DiMrB : Inport
  DiMrC : Inport  Port=2
  DiMrA : Inport  Port=3
  Constant2 : Constant  Value=-Lms
  Dot Product{,1..3} (4 alike) : DotProduct  InputSameDT=on  OutDataTypeStr=Inherit: Inherit via internal rule
  Sum : Sum  Inputs=|++
  Sum1 : Sum  Inputs=|++
  Trigonometric Function : Trigonometry  Operator=cos
  Trigonometric Function1 : Trigonometry  Operator=cos
  Trigonometric Function2 : Trigonometry  Operator=cos
  phi1 : Constant  Value=thetar
  phi2 = thetar + 2*pi/3 : Constant  Value=thetar + 2*pi/3
  phi3 = thetar - 2*pi/3 : Constant  Value=thetar - 2*pi/3
  F2B : Outport
  wires:
  Dot Product2/1 -> F2B/1
  Constant2/1 -> Dot Product2/2
  DiMrA/1 -> Dot Product1/2
  DiMrB/1 -> Dot Product/2
  phi1/1 -> Trigonometric Function/1
  Trigonometric Function2/1 -> Dot Product1/1  "cos(phi3)"
  phi2 = thetar + 2*pi/3/1 -> Trigonometric Function1/1
  Trigonometric Function/1 -> Dot Product/1  "cos(phi1)"
  phi3 = thetar - 2*pi/3/1 -> Trigonometric Function2/1
  Trigonometric Function1/1 -> Dot Product3/1  "cos(phi2)"
  Sum1/1 -> Dot Product2/1
  DiMrC/1 -> Dot Product3/2
  Dot Product1/1 -> Sum1/2
  Dot Product3/1 -> Sum/2
  Dot Product/1 -> Sum/1
  Sum/1 -> Sum1/1

== system blocos/wr/Subsystem/Disc/F1A1 ==
  DiMsA : Inport
  DiMsB : Inport  Port=2
  Constant : Constant  Value=Lms/2
  Dot Product : DotProduct  InputSameDT=on  OutDataTypeStr=Inherit: Inherit via internal rule
  Sum : Sum  Inputs=|++
  F1C : Outport
  wires:
  Constant/1 -> Dot Product/1
  Dot Product/1 -> F1C/1
  Sum/1 -> Dot Product/2
  DiMsB/1 -> Sum/2
  DiMsA/1 -> Sum/1

== system blocos/wr/Subsystem/Disc/F2A 1 ==
  DiMrC : Inport
  DiMrA : Inport  Port=2
  DiMrB : Inport  Port=3
  Constant2 : Constant  Value=-Lms
  Dot Product{,1..3} (4 alike) : DotProduct  InputSameDT=on  OutDataTypeStr=Inherit: Inherit via internal rule
  Sum : Sum  Inputs=|++
  Sum1 : Sum  Inputs=|++
  Trigonometric Function : Trigonometry  Operator=cos
  Trigonometric Function1 : Trigonometry  Operator=cos
  Trigonometric Function2 : Trigonometry  Operator=cos
  phi1 : Constant  Value=thetar
  phi2 = thetar + 2*pi/3 : Constant  Value=thetar + 2*pi/3
  phi3 = thetar - 2*pi/3 : Constant  Value=thetar - 2*pi/3
  F2C : Outport
  wires:
  Dot Product2/1 -> F2C/1
  Constant2/1 -> Dot Product2/2
  DiMrB/1 -> Dot Product1/2
  DiMrC/1 -> Dot Product/2
  phi1/1 -> Trigonometric Function/1
  Trigonometric Function2/1 -> Dot Product1/1  "cos(phi3)"
  phi2 = thetar + 2*pi/3/1 -> Trigonometric Function1/1
  Trigonometric Function/1 -> Dot Product/1  "cos(phi1)"
  phi3 = thetar - 2*pi/3/1 -> Trigonometric Function2/1
  Trigonometric Function1/1 -> Dot Product3/1  "cos(phi2)"
  Sum1/1 -> Dot Product2/1
  DiMrA/1 -> Dot Product3/2
  Dot Product1/1 -> Sum1/2
  Dot Product3/1 -> Sum/2
  Dot Product/1 -> Sum/1
  Sum/1 -> Sum1/1

== system blocos/wr/Subsystem5/Subsystem2/Subsystem1 ==
  Constant10 : Constant  Value=f
  Constant11 : Constant  Value=60
  Constant4 : Constant  Value=2
  Constant7 : Constant  Value=pi
  Constant8 : Constant  Value=polos
  Constant9 : Constant  Value=120
  Divide1 : Product  Inputs=*/
  Divide2 : Product  Inputs=*/
  Dot Product1 : DotProduct  InputSameDT=on  OutDataTypeStr=Inherit: Inherit via internal rule
  Dot Product5 : DotProduct  InputSameDT=on  OutDataTypeStr=Inherit: Inherit via internal rule
  Dot Product6 : DotProduct  InputSameDT=on  OutDataTypeStr=Inherit: Inherit via internal rule
  omega_1 : Outport
  wires:
  Constant9/1 -> Dot Product6/1
  Constant10/1 -> Dot Product6/2
  Constant7/1 -> Dot Product1/2
  Constant8/1 -> Divide2/2
  Dot Product6/1 -> Divide2/1
  Constant4/1 -> Dot Product1/1
  Dot Product5/1 -> omega_1/1
  Divide1/1 -> Dot Product5/2
  Dot Product1/1 -> Dot Product5/1
  Constant11/1 -> Divide1/2
  Divide2/1 -> Divide1/1
